simulink model "SPHERE_model2"  (R2020a)
settings: Solver=ode4  StartTime=0.0  StopTime=100  FixedStep=0.001  RelTol=1e-3
values from neighbouring files (symbols this model uses):
  delay_r = 0.05    [Initial_script.m]    (also in Initial_script_test.m; Initial_script_test2.m)
  K = 25.937    [Initial_script.m]    (also in Initial_script_test.m; Initial_script_test2.m)
  L = -[ M2*l*(-2*l + R) - 2*J2, 0, -2*M2*l*g ]    [Initial_script.m]    (also in Initial_script_test.m; Initial_script_test2.m)
  M = [ J1 + 2*J2 + M1*R^2 + M2*(2*l^2 - 3*R*l + R^2), -Tv, 2*l*g*M2 ]    [Initial_script.m]    (also in Initial_script_test.m; Initial_script_test2.m)
  Smax = 502    [Initial_script.m]    (also in Initial_script_test.m; Initial_script_test2.m)
  Smin = -480    [Initial_script.m]    (also in Initial_script_test.m; Initial_script_test2.m)
  Top = 0.015    [Initial_script.m]    (also in Initial_script_test.m; Initial_script_test2.m)
libraries: simulink x1
settings Model: Creator=Adrian  LastModifiedBy=Adrian

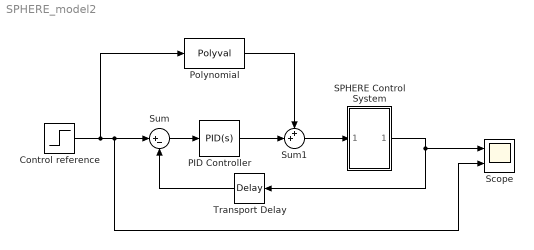
== system SPHERE_model2 ==
  Control reference : Step  Time=5  After=15  SampleTime=0
  PID Controller : simulink/Continuous/PID Controller  Controller=PID  Form=Parallel  TimeDomain=Continuous-time  UseExternalTs=off  SampleTime=-1  IntegratorMethod=Forward Euler  FilterMethod=Forward Euler  ControllerParametersSource=internal  P=0  I=0.137762209587736  D=0  UseFilter=on  N=100  TunerSelectOption=Transfer Function Based (PID Tuner App)  InitialConditionSource=internal  InitialConditionForIntegrator=0  InitialConditionForFilter=0  DifferentiatorICPrevScaledInput=0  ExternalReset=none  TrackingMode=off  Kt=1  LimitOutput=off  UpperSaturationLimit=inf  LowerSaturationLimit=-inf  LinearizeAsGain=on  AntiWindupMode=none  Kb=1  POutMin=[]  POutMax=[]  IOutMin=[]  IOutMax=[]  DOutMin=[]  DOutMax=[]  NOutMin=[]  NOutMax=[]  SumOutMin=[]  SumOutMax=[]  SaturationOutMin=[]  SaturationOutMax=[]  PParamMin=[]  PParamMax=[]  IParamMin=[]  IParamMax=[]  DParamMin=[]  DParamMax=[]  NParamMin=[]  NParamMax=[]  KbParamMin=[]  KbParamMax=[]  KtParamMin=[]  KtParamMax=[]  KbOutMin=[]  KbOutMax=[]  KtOutMin=[]  KtOutMax=[]  IntegratorOutMin=[]  IntegratorOutMax=[]  FilterOutMin=[]  FilterOutMax=[]  SumI1OutMin=[]  SumI1OutMax=[]  SumI2OutMin=[]  SumI2OutMax=[]  SumI3OutMin=[]  SumI3OutMax=[]  SumI4OutMin=[]  SumI4OutMax=[]  SumDOutMin=[]  SumDOutMax=[]  DifferentiatorOutMin=[]  DifferentiatorOutMax=[]  FilterDiffOutCoefMin=[]  FilterDiffOutCoefMax=[]  ReciprocalOutMin=[]  ReciprocalOutMax=[]  SumDenOutMin=[]  SumDenOutMax=[]  SumNumOutMin=[]  SumNumOutMax=[]  DivideOutMin=[]  DivideOutMax=[]  UdiffTsProdOutMin=[]  UdiffTsProdOutMax=[]  NTsProdOutMin=[]  NTsProdOutMax=[]  UintegralTsProdOutMin=[]  UintegralTsProdOutMax=[]  UngainTsProdOutMin=[]  UngainTsProdOutMax=[]  IntegratorContinuousStateAttributes=''  IntegratorStateMustResolveToSignalObject=off  IntegratorRTWStateStorageClass=Auto  FilterContinuousStateAttributes=''  FilterStateMustResolveToSignalObject=off  FilterRTWStateStorageClass=Auto  ParallelPVariant=InternalParameters  IdealPVariant=Disabled  IVariant=InternalParameters  DVariant=InternalParameters  IntegratorVariant=Continuous  SatVariant=Disabled  AWVariant=Passthrough  PCopyVariant=Disabled  TRVariant=Disabled  FdbkBlocksVariant=Forward  IdealPFdbkVariant=Disabled  SatFdbkVariant=Disabled  DerivativeFilterVariant=ContFilter  NVariant=InternalParameters  NCopyVariant=Disabled  FilterICVariant=InternalICsFilter  IntegratorICVariant=InternalICs  ExternalResetVariant=Disabled  TRSumVariant=Passthrough  SumFdbkVariant=Disabled  SumVariant=Sum_PID  TsampFilterVariant=InternalTs  TsampNgainVariant=Passthrough  TsampIntegralVariant=Passthrough
  Polynomial : Polyval  Coefs=[0.000325 0.001274 1.044515 0]
  SPHERE Control System : Subsystem
  Scope : Scope  NumInputPorts=2
  Sum : Sum  Inputs=|+-
  Sum1 : Sum  Inputs=++|
  Transport Delay : TransportDelay  DelayTime=delay_r
  wires:
  Control reference/1 -> Polynomial/1, Scope/2, Sum/1
  Sum/1 -> PID Controller/1
  SPHERE Control System/1(Out1) -> Transport Delay/1, Scope/1
  Sum1/1 -> SPHERE Control System/1(In1)
  PID Controller/1 -> Sum1/2
  Polynomial/1 -> Sum1/1
  Transport Delay/1 -> Sum/2

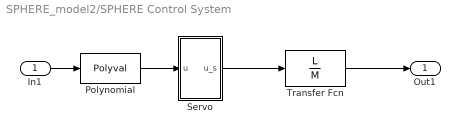
== system SPHERE_model2/SPHERE Control System ==
  In1 : Inport
  Polynomial : Polyval  Coefs=[-0.000067 -0.000287 0.871698 0]
  Servo : Subsystem
  Transfer Fcn : TransferFcn  Numerator=L  Denominator=M
  Out1 : Outport
  wires:
  Transfer Fcn/1 -> Out1/1
  In1/1 -> Polynomial/1
  Servo/1(u_s) -> Transfer Fcn/1
  Polynomial/1 -> Servo/1(u)

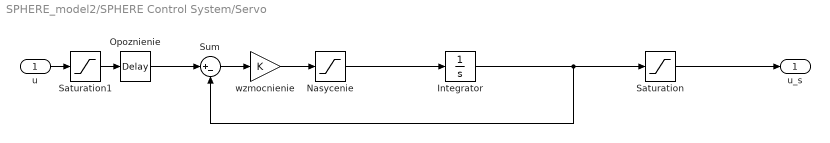
== system SPHERE_model2/SPHERE Control System/Servo ==
  u : Inport
  Integrator : Integrator
  Nasycenie : Saturate  UpperLimit=Smax  LowerLimit=Smin
  Opoznienie : TransportDelay  DelayTime=Top
  Saturation : Saturate  UpperLimit=60  LowerLimit=-60
  Saturation1 : Saturate  UpperLimit=60  LowerLimit=-60
  Sum : Sum  Inputs=|+-
  wzmocnienie : Gain  Gain=K
  u_s : Outport
  wires:
  Sum/1 -> wzmocnienie/1
  Integrator/1 -> Saturation/1, Sum/2
  wzmocnienie/1 -> Nasycenie/1
  Opoznienie/1 -> Sum/1
  Nasycenie/1 -> Integrator/1
  u/1 -> Saturation1/1
  Saturation/1 -> u_s/1
  Saturation1/1 -> Opoznienie/1
